simulink model "lab07"  (Simulink 10.3)
settings: Solver=VariableStepAuto  StartTime=0.0  StopTime=10.0  RelTol=1e-3
values from neighbouring files (symbols this model uses):
  A = [0 -17.7992575906 0 53.9371442139 1 -0.948653198653 0 0 0 15.9252369398 0 -18.56132406 ... (16 elements, 4x4)]    [lab03.mat]    (also in lab04.mat; lab05.mat = [25.4537620431 151.732816054 4.23886174535 50.4259963467]; lab06.mat = [25.4537620431 151.732816054 4.23886174535 50.4259963467]; lab07.mat = [0 -14.3493565507 0 286.595224124 1 -0.399597627389 0 0 0 3.)
  B = [0 6.73132472896 0 -7.64415309154]    [lab03.mat]    (also in lab04.mat; lab05.mat; lab06.mat; lab07.mat = [0 -969.89803323 0 15100.0389508])
  C = [0 0 1 0]    [lab03.mat]    (also in lab04.mat; lab05.mat; lab06.mat; lab07.mat = [1 0 0 0])
  C2 = [0 0 1 0]    [lab07.mat]
  D = 0    [lab03.mat]    (also in lab04.mat; lab05.mat; lab07.mat; matlab.mat)
  K = [0.240786866042 0.0805524158457 0.036570221416 0.00667411383528]    [lab07.mat]
  k_pf = 1    [lab02.mat]    (also in lab03.mat; lab04.mat; lab05.mat; lab06.mat)
settings Model: Creator=kisdev  LastModifiedBy=kisdev
settings SolverCC: AlgebraicLoopSolver=Auto
settings DataIOCC: SaveFormat=Dataset  SignalLoggingSaveFormat=Dataset  ReturnWorkspaceOutputs=on
settings OptimizationCC: ExpressionDepthLimit=128  LifeSpan=auto
settings DebuggingCC: UnderspecifiedInitializationDetection=Simplified  MergeDetectMultiDrivingBlocksExec=error  FcnCallInpInsideContextMsg=error  StateNameClashWarn=none  SFUnexpectedBacktrackingDiag=error  SFNoUnconditionalDefaultTransitionDiag=error  SFExecutionAtInitializationDiag=warning  SFMachineParentedDataDiag=error  ArithmeticOperatorsInVariantConditions=error
settings HardwareCC: ProdBitPerPointer=64  ProdBitPerSizeT=64  ProdBitPerPtrDiffT=64  ProdLargestAtomicFloat=Float  ProdIntDivRoundTo=Zero  ProdEndianess=LittleEndian  ProdWordSize=64  ProdHWDeviceType=Intel->x86-64 (Windows64)
settings ModelReferenceCC: PropagateSignalLabelsOutOfModel=on
settings SFSimCC: SimUseLocalCustomCode=on  CustomCodeUndefinedFunction=FilterOut
settings RTWCC: RTWUseLocalCustomCode=on
settings CodeAppCC: StateflowObjectComments=off
settings GRTTargetCC: TargetLangStandard=C99 (ISO)  CombineOutputUpdateFcns=on  GRTInterface=off
settings ConfigComp: CovMetricSettings=dwe  CovSaveCumulativeToWorkspaceVar=off  CovSaveSingleToWorkspaceVar=off  CovExternalEMLEnable=on

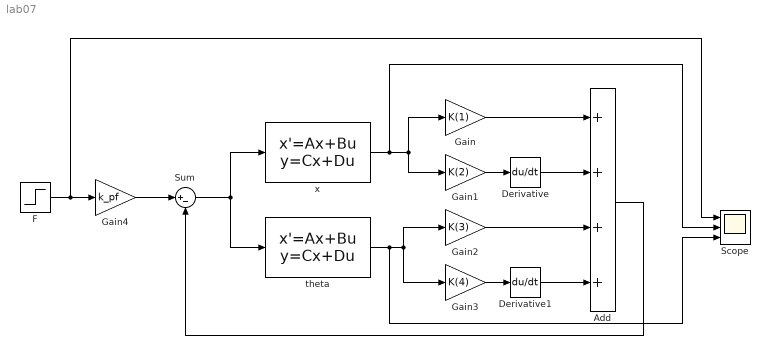
== system lab07 ==
  Add : Sum  Inputs=++++
  Derivative : Derivative
  Derivative1 : Derivative
  F : Step  SampleTime=0
  Gain : Gain  Gain=K(1)
  Gain1 : Gain  Gain=K(2)
  Gain2 : Gain  Gain=K(3)
  Gain3 : Gain  Gain=K(4)
  Gain4 : Gain  Gain=k_pf
  Scope : Scope  NumInputPorts=3
  Sum : Sum  Inputs=|+-
  theta : StateSpace  A=A  B=B  C=C2  D=D  InitialCondition=0
  x : StateSpace  A=A  B=B  C=C  D=D  InitialCondition=0
  wires:
  x/1 -> Scope/2, Gain/1, Gain1/1
  theta/1 -> Scope/3, Gain2/1, Gain3/1
  Gain1/1 -> Derivative/1
  Gain3/1 -> Derivative1/1
  Gain/1 -> Add/1
  Derivative/1 -> Add/2
  Gain2/1 -> Add/3
  Derivative1/1 -> Add/4
  Add/1 -> Sum/2
  Sum/1 -> x/1, theta/1
  Gain4/1 -> Sum/1
  F/1 -> Scope/1, Gain4/1
